simulink model "gm_uz_ssi_interface_2023a"  (R2023a)
settings: Solver=FixedStepDiscrete  StartTime=0.0  StopTime=0.0025  RelTol=1e-3
undefined symbols (not defined in the file or in its folder): binary_or_gray, bit_sum, delay_first_clk_on_off, f_ADC, f_clock, PLL, ssi_clk_divider, ssi_encoder_bit_width_multi_turn, ssi_encoder_bit_width_single_turn, ssi_encoder_number_of_status_bits, t_ADC, t_clock
libraries: hdlmdlgenlib x111, hdlsllib x62, simulink x27, simulink_extras x7
(part 4 of 4)

== system gm_uz_ssi_interface_2023a/uz_ssi_interface/position_to_speed_pll/Sine HDL Optimized1/sincos hdl/sin_hdl ==
  note: (C) 2016 Mathworks, Inc
  In1 : Inport  OutDataTypeStr=fixdt(1, 27, 20)  SampleTime=1e-08
  Amp50 : Sum  Inputs=+-  AccumDataTypeStr=fixdt(1, 28, 27)  OutDataTypeStr=fixdt(1, 28, 27)  SampleTime=1e-08
  CastU16En2 : DataTypeConversion  OutDataTypeStr=fixdt(0, 10, 0)  ConvertRealWorld=Stored Integer (SI)  SampleTime=1e-08  SaturateOnIntegerOverflow=off  RndMeth=Floor
  CastU16En3 : DataTypeConversion  OutDataTypeStr=fixdt(0, 10, 0)  ConvertRealWorld=Stored Integer (SI)  SampleTime=1e-08  RndMeth=Floor
  CastU16En4 : DataTypeConversion  OutDataTypeStr=fixdt(0, 11, 0)  SampleTime=1e-08  SaturateOnIntegerOverflow=off  RndMeth=Floor
  LTEp25 : RelationalOperator  Operator=<=  OutDataTypeStr=boolean  SampleTime=1e-08  InputSameDT=off
  LTEp50 : RelationalOperator  Operator=<=  OutDataTypeStr=boolean  SampleTime=1e-08  InputSameDT=off
  Look-Up Table : Lookup_n-D  NumberOfTableDimensions=1  BreakpointsForDimension1="fi(\"numerictype\",numerictype(0,10,0),\"fimath\",fimath(\"RoundingMethod\", \"Floor\",\"OverflowAction\", \"Wrap\",\"ProductMode\",\"FullPrecision\",\"SumMode\",\"FullPrecision\"),\"Value\",\"[0 1 2 3 4 5 6 7 8 9 10 11 12 13 14 15 16 17 18 19 20 21 22 23 24 25 26 27 28 29 30 31 32 33 34 35 36 37 38 39 40 41 42 43 44 45 46 47 48 49 50 51 52 53 54 55 56 57 58 59 60 61 62 63 64 65 66 67 68 69 70 71 72 73 74 75 76 77 78 79 80 81 82 83 84 85 86 87 88 89 90 91 92 93 94 95 96 97 98 99 100 101 102 103 104 105 106 107 108 109 110 111 112 113 114 115 116 117 118 119 120 121 122 123 124 125 126 127 128 129 130 131 132 133 134 135 136 137 138 139 140 141 142 143 144 145 146 147 148 149 150 151 152 153 154 155 156 157 158 159 160 161 162 163 164 165 166 167 168 169 170 171 172 173 174 175 176 177 178 179 180 181 182 183 184 185 186 187 188 189 190 191 192 193 194 195 196 197 198 199 200 201 202 203 204 205 206 207 208 209 210 211 212 213 214 215 216 217 218 219 220 221 222 223 224 225 226 227 228 229 230 231 232 233 234 235 236 237 238 239 240 241 242 243 244 245 246 247 248 249 250 251 252 253 254 255]\")"  Table="reshape(fi(\"numerictype\",numerictype(1,27,20),\"fimath\",fimath(\"RoundingMethod\", \"Floor\",\"OverflowAction\", \"Wrap\",\"ProductMode\",\"FullPrecision\",\"SumMode\",\"FullPrecision\"),\"Value\",\"[0;0.0061359405517578125;0.012271881103515625;0.01840686798095703125;0.02454090118408203125;0.03067493438720703125;0.03680706024169921875;0.042938232421875;0.04906749725341796875;0.055194854736328125;0.06132030487060546875;0.06744384765625;0.0735645294189453125;0.07968235015869140625;0.08579730987548828125;0.0919094085693359375;0.0980167388916015625;0.10412120819091796875;0.11022186279296875;0.11631870269775390625;0.12241077423095703125;0.128498077392578125;0.1345806121826171875;0.14065837860107421875;0.1467304229736328125;0.15279674530029296875;0.15885829925537109375;0.164913177490234375;0.17096233367919921875;0.1770038604736328125;0.18303966522216796875;0.18906879425048828125;0.19509029388427734375;0.20110416412353515625;0.207111358642578125;0.2131099700927734375;0.2191009521484375;0.2250843048095703125;0.2310581207275390625;0.23702335357666015625;0.24298000335693359375;0.248928070068359375;0.2548656463623046875;0.2607936859130859375;0.26671314239501953125;0.27262115478515625;0.27851963043212890625;0.28440761566162109375;0.2902851104736328125;0.29615116119384765625;0.302005767822265625;0.307849884033203125;0.31368160247802734375;0.3195018768310546875;0.32531070709228515625;0.3311061859130859375;0.33689022064208984375;0.3426609039306640625;0.34841823577880859375;0.35416316986083984375;0.35989475250244140625;0.36561298370361328125;0.3713169097900390625;0.37700748443603515625;0.38268375396728515625;0.38834476470947265625;0.39399242401123046875;0.399623870849609375;0.4052410125732421875;0.4108428955078125;0.4164295196533203125;0.42199993133544921875;0.427555084228515625;0.433094024658203125;0.4386157989501953125;0.444122314453125;0.449611663818359375;0.4550838470458984375;0.4605388641357421875;0.465976715087890625;0.47139644622802734375;0.47679901123046875;0.4821834564208984375;0.48754978179931640625;0.49289798736572265625;0.4982280731201171875;0.5035381317138671875;0.50883007049560546875;0.514102935791015625;0.51935577392578125;0.52458953857421875;0.52980327606201171875;0.5349979400634765625;0.54017162322998046875;0.54532527923583984375;0.55045795440673828125;0.5555706024169921875;0.56066131591796875;0.56573200225830078125;0.57078075408935546875;0.57580852508544921875;0.580814361572265625;0.5857982635498046875;0.59075927734375;0.595699310302734375;0.600616455078125;0.605510711669921875;0.61038303375244140625;0.61523151397705078125;0.62005710601806640625;0.62485980987548828125;0.629638671875;0.6343936920166015625;0.63912487030029296875;0.6438312530517578125;0.64851474761962890625;0.65317249298095703125;0.657806396484375;0.66241550445556640625;0.66699981689453125;0.67155933380126953125;0.67609310150146484375;0.6806011199951171875;0.6850833892822265625;0.689540863037109375;0.6939716339111328125;0.69837665557861328125;0.702754974365234375;0.70710659027099609375;0.71143245697021484375;0.7157306671142578125;0.72000217437744140625;0.724246978759765625;0.7284641265869140625;0.732654571533203125;0.73681640625;0.7409515380859375;0.7450580596923828125;0.7491359710693359375;0.7531871795654296875;0.75720882415771484375;0.76120281219482421875;0.765167236328125;0.76910305023193359375;0.77301025390625;0.77688884735107421875;0.7807369232177734375;0.78455638885498046875;0.78834629058837890625;0.79210662841796875;0.79583644866943359375;0.79953765869140625;0.8032073974609375;0.80684757232666015625;0.8104572296142578125;0.81403636932373046875;0.817584991455078125;0.821102142333984375;0.82458972930908203125;0.828044891357421875;0.83146953582763671875;0.83486270904541015625;0.8382244110107421875;0.8415546417236328125;0.84485340118408203125;0.84812068939208984375;0.85135555267333984375;0.85455799102783203125;0.8577289581298828125;0.860866546630859375;0.86397266387939453125;0.867046356201171875;0.870086669921875;0.8730945587158203125;0.8760700225830078125;0.87901210784912109375;0.88192081451416015625;0.88479709625244140625;0.8876399993896484375;0.89044857025146484375;0.8932247161865234375;0.89596652984619140625;0.89867401123046875 ...(+1615 chars)]\"), [1  256])"  InterpMethod=Flat  ExtrapMethod=Clip  DiagnosticForOutOfRangeInput=Error  SampleTime=1e-08  OutDataTypeStr=fixdt(1, 27, 20)
  Negate : UnaryMinus  SampleTime=1e-08
  PipelineRegister : Delay  DelayLength=double(1)  InitialCondition=0
  Point25 : Constant  Value=0.25  OutDataTypeStr=fixdt(0, 27, 27)  SampleTime=1e-08
  Point50 : Constant  Value=0.5  OutDataTypeStr=fixdt(0, 27, 27)  SampleTime=1e-08
  Positive : DataTypeConversion  OutDataTypeStr=fixdt(1,27,20)
  QuadHandle1 : Switch  Criteria=u2 ~= 0  Threshold=double(0)  OutDataTypeStr=fixdt(1, 28, 27)  SampleTime=1e-08  SaturateOnIntegerOverflow=off  InputSameDT=off
  QuadHandle2 : Switch  Criteria=u2 ~= 0  Threshold=double(0)  OutDataTypeStr=fixdt(0, 10, 10)  SampleTime=1e-08  SaturateOnIntegerOverflow=off  InputSameDT=off
  RAMDelayBalance : hdlmdlgenlib/Buffer
  Saturation : Saturate  UpperLimit="fi(0,0,10,0,\"hex\",\"0ff\")"  LowerLimit="fi(0,0,10,0,\"hex\",\"000\")"  SampleTime=1e-08  OutDataTypeStr=fixdt(0, 10, 0)
  SignCorrected : Switch  Criteria=u2 ~= 0  Threshold=double(0)  OutDataTypeStr=fixdt(1, 27, 20)  SampleTime=1e-08  SaturateOnIntegerOverflow=off  InputSameDT=off
  Switch : Switch  Criteria=u2 ~= 0  Threshold=double(0)  OutDataTypeStr=fixdt(0, 10, 0)  SampleTime=1e-08  SaturateOnIntegerOverflow=off  InputSameDT=off
  delayMatch : Delay  DelayLength=double(1)  InitialCondition=0
  insig : DataTypeConversion  OutDataTypeStr=fixdt(0, 10, 10)  SampleTime=1e-08  SaturateOnIntegerOverflow=off  RndMeth=Floor
  p50mA : Sum  Inputs=+-  AccumDataTypeStr=fixdt(1, 29, 27)  OutDataTypeStr=fixdt(1, 29, 27)  SampleTime=1e-08
  pow2switch : Constant  OutDataTypeStr=boolean  SampleTime=1e-08
  y : Outport  SampleTime=1e-08  InitialOutput=0
  wires:
  Amp50/1 -> QuadHandle1/3
  CastU16En2/1 -> CastU16En4/1
  CastU16En3/1 -> Switch/3, Saturation/1
  CastU16En4/1 -> CastU16En3/1
  LTEp25/1 -> QuadHandle2/2
  LTEp50/1 -> QuadHandle1/2, RAMDelayBalance/1
  PipelineRegister/1 -> Positive/1, Negate/1
  Negate/1 -> SignCorrected/3
  Point25/1 -> LTEp25/2
  Point50/1 -> p50mA/1, LTEp50/2, Amp50/2
  Positive/1 -> SignCorrected/1
  QuadHandle1/1 -> p50mA/2, QuadHandle2/1, LTEp25/1
  QuadHandle2/1 -> CastU16En2/1
  delayMatch/1 -> SignCorrected/2
  Saturation/1 -> Switch/1
  SignCorrected/1 -> y/1
  Switch/1 -> Look-Up Table/1
  insig/1 -> QuadHandle1/1, LTEp50/1, Amp50/1
  p50mA/1 -> QuadHandle2/3
  pow2switch/1 -> Switch/2
  In1/1 -> insig/1
  RAMDelayBalance/1 -> delayMatch/1
  Look-Up Table/1 -> PipelineRegister/1

== system gm_uz_ssi_interface_2023a/uz_ssi_interface/ssi_communication/sample_serial_ssi_data/Sample and Hold1/Model ==
  In : Inport  OutDataTypeStr=boolean  SampleTime=1e-08
  S : Inport  Port=2  OutDataTypeStr=boolean  SampleTime=1e-08
  Data Type Conversion : DataTypeConversion  OutDataTypeStr=boolean  SaturateOnIntegerOverflow=off  RndMeth=Floor
  IC=ic : UnitDelay  InitialCondition=ic  SampleTime=Ts  HasFrameUpgradeWarning=on
  Switch : Switch  Criteria=u2 ~= 0  SampleTime=Ts
  Out : Outport  SampleTime=1e-08
  wires:
  Data Type Conversion/1 -> Switch/2
  Switch/1 -> Out/1, IC=ic/1
  In/1 -> Switch/1
  S/1 -> Data Type Conversion/1
  IC=ic/1 -> Switch/3

== matlab function gm_uz_ssi_interface_2023a/uz_ssi_interface/position_to_speed_pll/fixed_point_floor/fixed_point_floor ==
  data: x input; y output
function y = fcn(x)
%#codegen
x_floor = bitsra(x, x.FractionLength);  % Shift right to remove fraction
x_floor = bitsll(x_floor, x.FractionLength);  % Shift left to restore scale

y = x_floor;

== matlab function gm_uz_ssi_interface_2023a/uz_ssi_interface/wrap_2pi_after_offset/fixed_point_floor/fixed_point_floor ==
  data: x input; y output
function y = fcn(x)
%#codegen
x_floor = bitsra(x, x.FractionLength);  % Shift right to remove fraction
x_floor = bitsll(x_floor, x.FractionLength);  % Shift left to restore scale

y = x_floor;

== matlab function gm_uz_ssi_interface_2023a/ssi_encoder/MATLAB Function ==
  data: u input; y output
function y = BinaryToGray(u)
%#codegen

y = bitxor(u,(bitshift(u,-1)));

== matlab function gm_uz_ssi_interface_2023a/uz_ssi_interface/wrap_2pi/fixed_point_floor/fixed_point_floor ==
  data: x input; y output
function y = fcn(x)
%#codegen
x_floor = bitsra(x, x.FractionLength);  % Shift right to remove fraction
x_floor = bitsll(x_floor, x.FractionLength);  % Shift left to restore scale

y = x_floor;
